simulink library "bus_stubs_template"  (R2016b)
settings: Solver=VariableStepAuto  StartTime=0.0  StopTime=10.0  RelTol=1e-3  EnableMultiTasking=on
settings Model: Creator=Jake  LastModifiedBy=bijan
settings DataIOCC: LimitDataPoints=on
settings OptimizationCC: LifeSpan=inf
settings DebuggingCC: AllowSymbolicDim=off  SFUnexpectedBacktrackingDiag=warning  SFNoUnconditionalDefaultTransitionDiag=warning  SFExecutionAtInitializationDiag=none
settings ModelReferenceCC: PropagateSignalLabelsOutOfModel=off
settings GRTTargetCC: TargetLangStandard=C89/C90 (ANSI)
settings ConfigComp: CovMetricSettings=dw  CovHtmlReporting=on  CovSaveCumulativeToWorkspaceVar=on  CovSaveSingleToWorkspaceVar=on  CovExternalEMLEnable=off

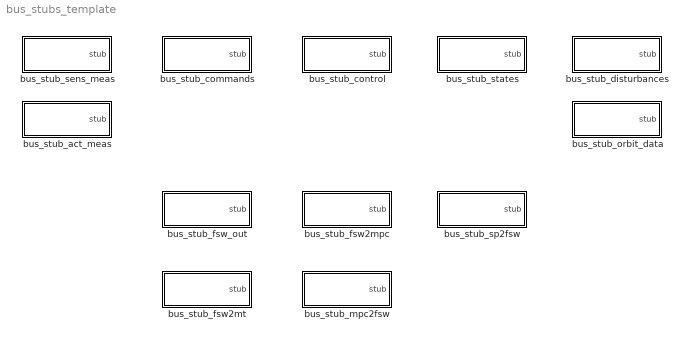
== system bus_stubs_template ==
  bus_stub_act_meas : Subsystem  mask(bus_stub_measurements){}
      mask help: Creates bus compliant with the measurements bus object.
      mask Help: Provides a zeroed bus which complies with the measurement bus object.
      mask DialogControl DescGroupVar Prompt: bus_stub_measurements
      mask DialogControl DescTextVar Prompt: Creates bus compliant with the measurements bus object.
  bus_stub_commands : Subsystem
      mask help: Creates bus compliant with actuatorCmd (actuator command) bus object.
      mask Help: Provides a zeroed bus which complies with the actuatorCmd bus object.
      mask DialogControl DescGroupVar Prompt: bus_stub_actCmd
      mask DialogControl DescTextVar Prompt: Creates bus compliant with actuatorCmd (actuator command) bus object.
  bus_stub_control : Subsystem  mask(bus_stub_actState){}
      mask help: Provides a zeroed bus which complies with the actuatorState bus object.
      mask Help: Provides a zeroed bus which complies with the actuatorState bus object.
      mask DialogControl DescGroupVar Prompt: bus_stub_actState
      mask DialogControl DescTextVar Prompt: Provides a zeroed bus which complies with the actuatorState bus object.
  bus_stub_disturbances : Subsystem  mask(bus_stub_env){}
      mask help: Creates bus compliant with the environment bus object.
      mask Help: Provides a zeroed bus which complies with the environment bus object.
      mask DialogControl DescGroupVar Prompt: bus_stub_env
      mask DialogControl DescTextVar Prompt: Creates bus compliant with the environment bus object.
  bus_stub_fsw2mpc : Subsystem
      mask help: Creates bus compliant with actuatorCmd (actuator command) bus object.
      mask Help: Provides a zeroed bus which complies with the actuatorCmd bus object.
      mask DialogControl DescGroupVar Prompt: bus_stub_actCmd
      mask DialogControl DescTextVar Prompt: Creates bus compliant with actuatorCmd (actuator command) bus object.
  bus_stub_fsw2mt : Subsystem
      mask help: Creates bus compliant with actuatorCmd (actuator command) bus object.
      mask Help: Provides a zeroed bus which complies with the actuatorCmd bus object.
      mask DialogControl DescGroupVar Prompt: bus_stub_actCmd
      mask DialogControl DescTextVar Prompt: Creates bus compliant with actuatorCmd (actuator command) bus object.
  bus_stub_fsw_out : Subsystem
      mask help: Creates bus compliant with actuatorCmd (actuator command) bus object.
      mask Help: Provides a zeroed bus which complies with the actuatorCmd bus object.
      mask DialogControl DescGroupVar Prompt: bus_stub_actCmd
      mask DialogControl DescTextVar Prompt: Creates bus compliant with actuatorCmd (actuator command) bus object.
  bus_stub_mpc2fsw : Subsystem
      mask help: Creates bus compliant with actuatorCmd (actuator command) bus object.
      mask Help: Provides a zeroed bus which complies with the actuatorCmd bus object.
      mask DialogControl DescGroupVar Prompt: bus_stub_actCmd
      mask DialogControl DescTextVar Prompt: Creates bus compliant with actuatorCmd (actuator command) bus object.
  bus_stub_orbit_data : Subsystem  mask(bus_stub_env){}
      mask help: Creates bus compliant with the environment bus object.
      mask Help: Provides a zeroed bus which complies with the environment bus object.
      mask DialogControl DescGroupVar Prompt: bus_stub_env
      mask DialogControl DescTextVar Prompt: Creates bus compliant with the environment bus object.
  bus_stub_sens_meas : Subsystem  mask(bus_stub_measurements){}
      mask help: Creates bus compliant with the measurements bus object.
      mask Help: Provides a zeroed bus which complies with the measurement bus object.
      mask DialogControl DescGroupVar Prompt: bus_stub_measurements
      mask DialogControl DescTextVar Prompt: Creates bus compliant with the measurements bus object.
  bus_stub_sp2fsw : Subsystem
      mask help: Creates bus compliant with actuatorCmd (actuator command) bus object.
      mask Help: Provides a zeroed bus which complies with the actuatorCmd bus object.
      mask DialogControl DescGroupVar Prompt: bus_stub_actCmd
      mask DialogControl DescTextVar Prompt: Creates bus compliant with actuatorCmd (actuator command) bus object.
  bus_stub_states : Subsystem  mask(bus_stub_state){}
      mask help: Creates bus compliant with the state bus object.
      mask Help: Provides a zeroed bus which complies with the state bus object.
      mask DialogControl DescGroupVar Prompt: bus_stub_state
      mask DialogControl DescTextVar Prompt: Creates bus compliant with the state bus object.

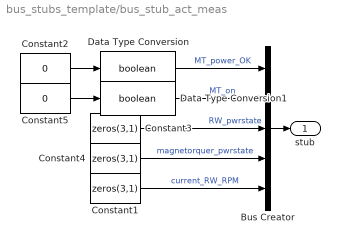
== system bus_stubs_template/bus_stub_act_meas ==
  Bus Creator : BusCreator  Inputs=5
  Constant1 : Constant  Value=zeros(3,1)
  Constant2 : Constant  Value=0
  Constant3 : Constant  Value=zeros(3,1)
  Constant4 : Constant  Value=zeros(3,1)
  Constant5 : Constant  Value=0
  Data Type Conversion : DataTypeConversion  OutDataTypeStr=boolean
  Data Type Conversion1 : DataTypeConversion  OutDataTypeStr=boolean
  stub : Outport  OutDataTypeStr=Bus: act_meas
  wires:
  Bus Creator/1 -> stub/1
  Constant4/1 -> Bus Creator/4  "magnetorquer_pwrstate"
  Constant3/1 -> Bus Creator/3  "RW_pwrstate"
  Constant1/1 -> Bus Creator/5  "current_RW_RPM"
  Constant2/1 -> Data Type Conversion/1
  Constant5/1 -> Data Type Conversion1/1
  Data Type Conversion/1 -> Bus Creator/1  "MT_power_OK"
  Data Type Conversion1/1 -> Bus Creator/2  "MT_on"

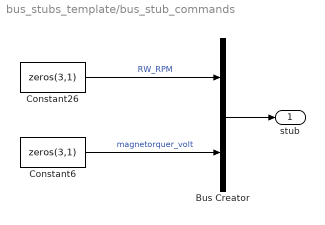
== system bus_stubs_template/bus_stub_commands ==
  Bus Creator : BusCreator  Inputs=2
  Constant26 : Constant  Value=zeros(3,1)
  Constant6 : Constant  Value=zeros(3,1)
  stub : Outport  OutDataTypeStr=Bus: commands
  wires:
  Bus Creator/1 -> stub/1
  Constant6/1 -> Bus Creator/2  "magnetorquer_volt"
  Constant26/1 -> Bus Creator/1  "RW_RPM"

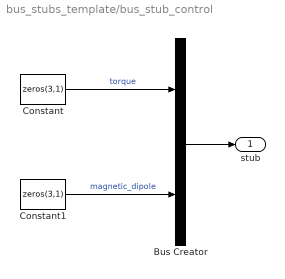
== system bus_stubs_template/bus_stub_control ==
  Bus Creator : BusCreator  Inputs=2
  Constant : Constant  Value=zeros(3,1)
  Constant1 : Constant  Value=zeros(3,1)
  stub : Outport  OutDataTypeStr=Bus: control
  wires:
  Bus Creator/1 -> stub/1
  Constant/1 -> Bus Creator/1  "torque"
  Constant1/1 -> Bus Creator/2  "magnetic_dipole"

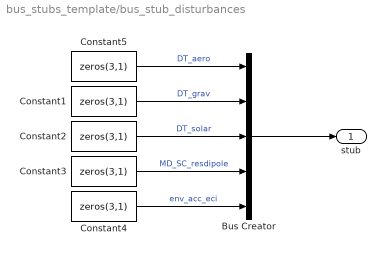
== system bus_stubs_template/bus_stub_disturbances ==
  Bus Creator : BusCreator  Inputs=5
  Constant{1..5} (5 alike) : Constant  Value=zeros(3,1)
  stub : Outport  OutDataTypeStr=Bus: disturbances
  wires:
  Bus Creator/1 -> stub/1
  Constant5/1 -> Bus Creator/1  "DT_aero"
  Constant1/1 -> Bus Creator/2  "DT_grav"
  Constant2/1 -> Bus Creator/3  "DT_solar"
  Constant3/1 -> Bus Creator/4  "MD_SC_resdipole"
  Constant4/1 -> Bus Creator/5  "env_acc_eci"

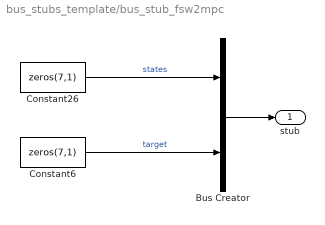
== system bus_stubs_template/bus_stub_fsw2mpc ==
  Bus Creator : BusCreator  Inputs=2
  Constant26 : Constant  Value=zeros(7,1)
  Constant6 : Constant  Value=zeros(7,1)
  stub : Outport  OutDataTypeStr=Bus: commands
  wires:
  Bus Creator/1 -> stub/1
  Constant6/1 -> Bus Creator/2  "target"
  Constant26/1 -> Bus Creator/1  "states"

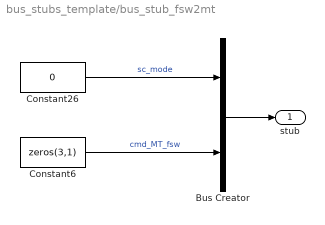
== system bus_stubs_template/bus_stub_fsw2mt ==
  Bus Creator : BusCreator  Inputs=2
  Constant26 : Constant  Value=0
  Constant6 : Constant  Value=zeros(3,1)
  stub : Outport  OutDataTypeStr=Bus: commands
  wires:
  Constant26/1 -> Bus Creator/1  "sc_mode"
  Constant6/1 -> Bus Creator/2  "cmd_MT_fsw"
  Bus Creator/1 -> stub/1

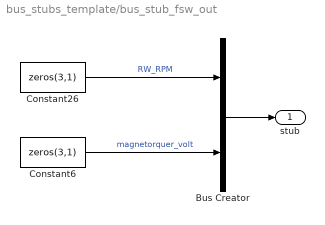
== system bus_stubs_template/bus_stub_fsw_out ==
  Bus Creator : BusCreator  Inputs=2
  Constant26 : Constant  Value=zeros(3,1)
  Constant6 : Constant  Value=zeros(3,1)
  stub : Outport  OutDataTypeStr=Bus: commands
  wires:
  Constant26/1 -> Bus Creator/1  "RW_RPM"
  Constant6/1 -> Bus Creator/2  "magnetorquer_volt"
  Bus Creator/1 -> stub/1

== system bus_stubs_template/bus_stub_mpc2fsw ==
  Bus Creator : BusCreator  Inputs=2
  Constant26 : Constant  Value=zeros(3,1)
  Constant6 : Constant  Value=0
  stub : Outport  OutDataTypeStr=Bus: mpc2fsw
  wires:
  Constant26/1 -> Bus Creator/1  "command"
  Constant6/1 -> Bus Creator/2  "status"
  Bus Creator/1 -> stub/1

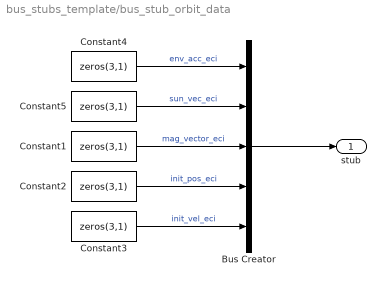
== system bus_stubs_template/bus_stub_orbit_data ==
  Bus Creator : BusCreator  Inputs=5
  Constant{1..5} (5 alike) : Constant  Value=zeros(3,1)
  stub : Outport  OutDataTypeStr=Bus: orbit_data
  wires:
  Constant3/1 -> Bus Creator/5  "init_vel_eci"
  Constant2/1 -> Bus Creator/4  "init_pos_eci"
  Constant1/1 -> Bus Creator/3  "mag_vector_eci"
  Constant5/1 -> Bus Creator/2  "sun_vec_eci"
  Bus Creator/1 -> stub/1
  Constant4/1 -> Bus Creator/1  "env_acc_eci"

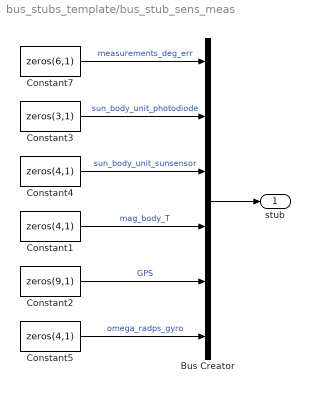
== system bus_stubs_template/bus_stub_sens_meas ==
  Bus Creator : BusCreator  Inputs=6
  Constant1 : Constant  Value=zeros(4,1)
  Constant2 : Constant  Value=zeros(9,1)
  Constant3 : Constant  Value=zeros(3,1)
  Constant4 : Constant  Value=zeros(4,1)
  Constant5 : Constant  Value=zeros(4,1)
  Constant7 : Constant  Value=zeros(6,1)
  stub : Outport  OutDataTypeStr=Bus: sens_meas
  wires:
  Constant3/1 -> Bus Creator/2  "sun_body_unit_photodiode"
  Constant4/1 -> Bus Creator/3  "sun_body_unit_sunsensor"
  Bus Creator/1 -> stub/1
  Constant1/1 -> Bus Creator/4  "mag_body_T"
  Constant2/1 -> Bus Creator/5  "GPS"
  Constant5/1 -> Bus Creator/6  "omega_radps_gyro"
  Constant7/1 -> Bus Creator/1  "measurements_deg_err"

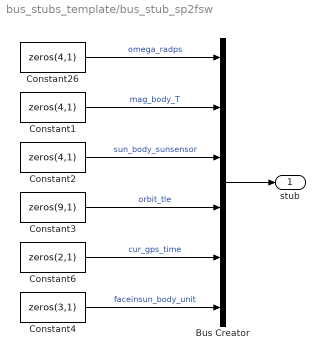
== system bus_stubs_template/bus_stub_sp2fsw ==
  Bus Creator : BusCreator  Inputs=6
  Constant1 : Constant  Value=zeros(4,1)
  Constant2 : Constant  Value=zeros(4,1)
  Constant26 : Constant  Value=zeros(4,1)
  Constant3 : Constant  Value=zeros(9,1)
  Constant4 : Constant  Value=zeros(3,1)
  Constant6 : Constant  Value=zeros(2,1)
  stub : Outport  OutDataTypeStr=Bus: commands
  wires:
  Bus Creator/1 -> stub/1
  Constant26/1 -> Bus Creator/1  "omega_radps"
  Constant1/1 -> Bus Creator/2  "mag_body_T"
  Constant2/1 -> Bus Creator/3  "sun_body_sunsensor"
  Constant3/1 -> Bus Creator/4  "orbit_tle"
  Constant6/1 -> Bus Creator/5  "cur_gps_time"
  Constant4/1 -> Bus Creator/6  "faceinsun_body_unit"

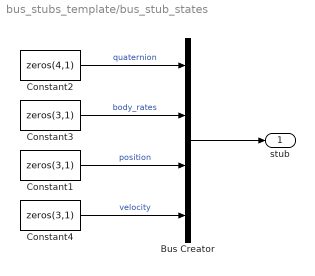
== system bus_stubs_template/bus_stub_states ==
  Bus Creator : BusCreator  Inputs=4
  Constant1 : Constant  Value=zeros(3,1)
  Constant2 : Constant  Value=zeros(4,1)
  Constant3 : Constant  Value=zeros(3,1)
  Constant4 : Constant  Value=zeros(3,1)
  stub : Outport  OutDataTypeStr=Bus: states
  wires:
  Bus Creator/1 -> stub/1
  Constant2/1 -> Bus Creator/1  "quaternion"
  Constant3/1 -> Bus Creator/2  "body_rates"
  Constant1/1 -> Bus Creator/3  "position"
  Constant4/1 -> Bus Creator/4  "velocity"
